simulink model "example_mpc_trajectory"  (R2015b)
settings: Solver=FixedStepAuto  StartTime=0.0  StopTime=50  FixedStep=Ts  RelTol=1e-3
InitFcn:
  | mpc_trajectory_data_callback
values from neighbouring files (symbols this model uses):
  Ts = 1    [example_mpc_cycle.m]
undefined symbols (not defined in the file or in its folder): sCoeffs, sPolyorder, sTimes
settings Model: Creator=Daniel  LastModifiedBy=mgreiff
settings SolverCC: AlgebraicLoopSolver=LineSearch

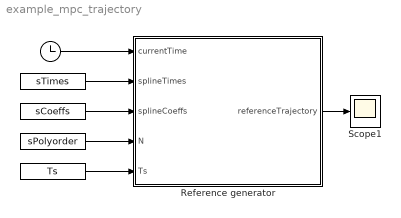
== system example_mpc_trajectory ==
  " " : Constant  Value=Ts
  "  " : Constant  Value=sPolyorder
  "   " : Constant  Value=sCoeffs
  "    " : Constant  Value=sTimes
  "      " : Clock
  Reference generator : MATLAB Function  TreatAsAtomicUnit=on
  Scope1 : Scope
  wires:
  "      "/1 -> Reference generator/1(currentTime)
  "    "/1 -> Reference generator/2(splineTimes)
  Reference generator/1(referenceTrajectory) -> Scope1/1
  "   "/1 -> Reference generator/3(splineCoeffs)
  "  "/1 -> Reference generator/4(N)
  " "/1 -> Reference generator/5(Ts)

== matlab function example_mpc_trajectory/Reference generator ==
  data: currentTime input; referenceTrajectory output; splineTimes input; splineCoeffs input; N input; Ts input
function referenceTrajectory = fcn(currentTime, splineTimes, splineCoeffs, N, Ts)
%#codegen

predHorizon = 4; % Number of points on the prediction horizon

times = currentTime + Ts.* (0:predHorizon-1);
referenceTrajectory = zeros(6,predHorizon);

for ii = 1:predHorizon
    % Finds the spline to evaluate
    T = times(ii);
    splineNumber = sum(splineTimes <=  T);

    % Treats the case when the time is outside the defined interval [t_0,t_s]
    if splineNumber == 0
        disp('Tried to evaluate spline before t_0, setting reference to the initial spline point.')
        T = splineTimes(1);
        splineNumber = 1;
    elseif T >= splineTimes(end)
        disp('Tried to evaluate spline after t_s, keeping position in terinal spline point')
        T = splineTimes(end);
        splineNumber = length(splineCoeffs(:,1))/(N + 1);
    end
    % Evaluates splines and stores data in referenceTrajectory
    for dim = 1:3
        startIndex = (N + 1) * (splineNumber - 1) + 1;
        endIndex = (N + 1) * splineNumber;
        poscoeff = splineCoeffs(startIndex:endIndex,dim);
        poscoeff = poscoeff(end:-1:1); % Reverses for polyval
        tt = T - splineTimes(splineNumber);

        % Position
        referenceTrajectory(dim,ii) = polyval(poscoeff,tt);

        % Velocity
        poscoeff(end) = [];
        velcoeff = (length(poscoeff):-1:1)'.*poscoeff; 
        referenceTrajectory(dim + 3,ii) = polyval(velcoeff,tt);
    end
end
